simulink model "Md62StEnCtrl"  (R2018b)
settings: Solver=FixedStepDiscrete  StartTime=0.0  StopTime=10.0  RelTol=1e-3
undefined symbols (not defined in the file or in its folder): data, KeSMSuFirstRwStBackPosDelta_Val, KeSMSuThrdRwCushFoldPosDelta_Val, KeSMSwAcsMd30PassStFldUpwdDnwdPos1_Val, KeSMSwAcsMd30PassStFrwdBkwdPos1_Val, KeSMSwAcsMd31PassStBkReclnUpwdDnwdPos1_Val, KeSMSwSeatBkLimitPos_Val, KeSMSwSeatBkLimitPosDelt_Val, PassStBkReclnEn_Clear, PassStBkReclnEn_Set, PassStCshnFldEn_Clear, PassStCshnFldEn_Set, PassStFwdBkwdEn_Clear, PassStFwdBkwdEn_Set, SecRwLtStBkReclnEn_Clear, SecRwLtStBkReclnEn_Set, SecRwLtStFwdBkwdEn_Clear, SecRwLtStFwdBkwdEn_Set, SecRwLtStLgrstInwdOtwdEn_Clear, SecRwLtStLgrstInwdOtwdEn_Set, SecRwLtStLgrstUpwdDnwdEn_Clear, SecRwLtStLgrstUpwdDnwdEn_Set, SecRwRtStBkReclnEn_Clear, SecRwRtStBkReclnEn_Set, SecRwRtStFwdBkwdEn_Clear, SecRwRtStFwdBkwdEn_Set, SecRwRtStLgrstInwdOtwdEn_Clear, SecRwRtStLgrstInwdOtwdEn_Set, SecRwRtStLgrstUpwdDnwdEn_Clear, SecRwRtStLgrstUpwdDnwdEn_Set, ThdRwLtStBkReclnEn_Clear, ThdRwLtStBkReclnEn_Set, ThdRwLtStCshnFldEn_Clear, ThdRwLtStCshnFldEn_Set, ThdRwLtStFwdBkwdEn_Clear, ThdRwLtStFwdBkwdEn_Set, ThdRwRtStBkReclnEn_Clear, ThdRwRtStBkReclnEn_Set, ThdRwRtStCshnFldEn_Clear, ThdRwRtStCshnFldEn_Set, ThdRwRtStFwdBkwdEn_Clear, ThdRwRtStFwdBkwdEn_Set, ZeroLEn_Clear, ZeroLEn_Set, ZeroREn_Clear, ZeroREn_Set
libraries: simulink x1
(part 3 of 3)

== system Md62StEnCtrl/Md62StEnCtrl_Cal_sys/Subsystem/ThdRwRtStFwdBkwd_Clear ==
  note: Delete block
  MdBitNum : Inport
  Action Port : ActionPort  ActionType=else
  ThdRwRtStFwdBkwdEn_Clear : FunctionCaller  FunctionPrototype=ThdRwRtStFwdBkwdEn_Clear(data)  InputArgumentSpecifications=uint8(1)
  wires:
  MdBitNum/1 -> ThdRwRtStFwdBkwdEn_Clear/1

== system Md62StEnCtrl/Md62StEnCtrl_Cal_sys/Subsystem/ThdRwRtStFwdBkwd_Set ==
  note: Delete block
  MdBitNum : Inport
  Action Port : ActionPort  ActionType=then
  ThdRwRtStFwdBkwdEn_Set : FunctionCaller  FunctionPrototype=ThdRwRtStFwdBkwdEn_Set(data)  InputArgumentSpecifications=uint8(1)
  wires:
  MdBitNum/1 -> ThdRwRtStFwdBkwdEn_Set/1

== system Md62StEnCtrl/Md62StEnCtrl_Cal_sys/Subsystem/ZeroL_Clear ==
  note: Delete block
  MdBitNum : Inport
  Action Port : ActionPort  ActionType=else
  ZeroLEn_Clear : FunctionCaller  FunctionPrototype=ZeroLEn_Clear(data)  InputArgumentSpecifications=uint8(1)
  wires:
  MdBitNum/1 -> ZeroLEn_Clear/1

== system Md62StEnCtrl/Md62StEnCtrl_Cal_sys/Subsystem/ZeroL_Set ==
  note: Delete block
  MdBitNum : Inport
  Action Port : ActionPort  ActionType=then
  ZeroLEn_Set : FunctionCaller  FunctionPrototype=ZeroLEn_Set(data)  InputArgumentSpecifications=uint8(1)
  wires:
  MdBitNum/1 -> ZeroLEn_Set/1

== system Md62StEnCtrl/Md62StEnCtrl_Cal_sys/Subsystem/ZeroR_Clear ==
  note: Delete block
  MdBitNum : Inport
  Action Port : ActionPort  ActionType=else
  ZeroREn_Clear : FunctionCaller  FunctionPrototype=ZeroREn_Clear(data)  InputArgumentSpecifications=uint8(1)
  wires:
  MdBitNum/1 -> ZeroREn_Clear/1

== system Md62StEnCtrl/Md62StEnCtrl_Cal_sys/Subsystem/ZeroR_Set ==
  note: Delete block
  MdBitNum : Inport
  Action Port : ActionPort  ActionType=then
  ZeroREn_Set : FunctionCaller  FunctionPrototype=ZeroREn_Set(data)  InputArgumentSpecifications=uint8(1)
  wires:
  MdBitNum/1 -> ZeroREn_Set/1

== stateflow chart Md62StEnCtrl/Md62StEnCtrl_Cal_sys/Subsystem/Chart ==
  (default) -> (junction 20) : {
      | PassStBkReclnEn = 0;
      | PassStCshnFldEn = 0;
      | PassStFwdBkwdEn=0;
      | SecRwLtStBkReclnEn=0;
      | SecRwLtStFwdBkwdEn=0;
      | SecRwLtStLgrstInwdOtwdEn=0;
      | SecRwLtStLgrstUpwdDnwdEn=0;
      | SecRwRtStBkReclnEn=0;
      | SecRwRtStFwdBkwdEn=0;
      | SecRwRtStLgrstInwdOtwdEn=0;
      | SecRwRtStLgrstUpwdDnwdEn=0;
      | ThdRwLtStBkReclnEn=0;
      | ThdRwLtStCshnFldEn=0;
      | ThdRwLtStFwdBkwdEn=0;
      | ThdRwRtStBkReclnEn=0;
      | ThdRwRtStCshnFldEn=0;
      | ThdRwRtStFwdBkwdEn=0;
      | ZeroLEn=0;
      | ZeroREn=0;
      | PassStFwdBkwdFailflg = 0;
      | PassStCshnFldFailflg = 0;
      | }
  (junction 20) -> (junction 22) [order 1] : [!Stage1SecRwDone]
  (junction 22) -> (junction 26) [order 1] : [Md61ThdRwNotNeedFldOpn]
  (junction 20) -> (junction 44) [order 2]
  (junction 22) -> (junction 37) [order 2]
  (junction 26) -> (junction 28) : {
      | SecRwRtStLgrstInwdOtwdEn=1;
      | SecRwRtStLgrstUpwdDnwdEn=1;
      | }
  (junction 37) -> (junction 39) [order 1] : [Md61ThdRwLtStNotNeedFldOpn]
  (junction 39) -> (junction 499) [order 1] : [!SecRwRtStBkReclnStgDone ||...
      | !SecRwRtStLgrstOtwdInwdStgDone ||...
      | !SecRwRtStLgrstUpwdDnwdStgDone]
  (junction 44) -> (junction 46) [order 1] : [ThdRwLtNeedFld]
  (junction 46) -> (junction 52) [order 1] : [!ThdRwLtStBkReclnStgDone||!ThdRwLtStFwdBkwdStgDone]
  (junction 37) -> (junction 504) [order 2]
  (junction 39) -> (junction 41) [order 2] : {
      | SecRwRtStFwdBkwdEn=1;
      | }
  (junction 499) -> (junction 501) : {SecRwRtStLgrstInwdOtwdEn=1;
      | SecRwRtStLgrstUpwdDnwdEn=1;
      | SecRwRtStBkReclnEn=1;}
  (junction 44) -> (junction 71) [order 2]
  (junction 46) -> (junction 64) [order 2]
  (junction 52) -> (junction 56) : {
      | ThdRwLtStBkReclnEn = 1;
      | ThdRwLtStFwdBkwdEn=1;
      | }
  (junction 64) -> (junction 66) [order 1] : [!ThdRwLtStCshnFldStgDone]
  (junction 64) -> (junction 54) [order 2]
  (junction 66) -> (junction 68) : {
      | ThdRwLtStCshnFldEn=1;
      | }
  (junction 504) -> (junction 506) [order 1] : [!SecRwRtStBkReclnStgDone ||...
      | !SecRwRtStLgrstOtwdInwdStgDone ||...
      | !SecRwRtStLgrstUpwdDnwdStgDone]
  (junction 504) -> (junction 510) [order 2] : {SecRwRtStFwdBkwdEn=1;}
  (junction 506) -> (junction 508) : {SecRwRtStLgrstInwdOtwdEn=1;
      | SecRwRtStLgrstUpwdDnwdEn=1;
      | SecRwRtStBkReclnEn=1;}
  (junction 68) -> (junction 54)
  (junction 56) -> (junction 68)
  (junction 54) -> (junction 71)
  (junction 71) -> (junction 74)
  (junction 508) -> (junction 510)
  (junction 74) -> (junction 76) [order 1] : [ThdRwLtNeedOpn]
  (junction 76) -> (junction 78) [order 1] : [!ThdRwLtStCshnFldStgDone]
  (junction 510) -> (junction 513)
  (junction 74) -> (junction 92) [order 2]
  (junction 76) -> (junction 84) [order 2]
  (junction 78) -> (junction 80) : {
      | ThdRwLtStCshnFldEn=1;
      | }
  (junction 84) -> (junction 87) [order 1] : [!ThdRwLtStBkReclnStgDone||!ThdRwLtStFwdBkwdStgDone]
  (junction 84) -> (junction 82) [order 2]
  (junction 87) -> (junction 89) : {
      | ThdRwLtStBkReclnEn = 1;
      | ThdRwLtStFwdBkwdEn=1;
      | }
  (junction 513) -> (junction 515) [order 1] : [!SecRwLtStBkReclnStgDone ||...
      | !SecRwLtStLgrstOtwdInwdStgDone ||...
      | !SecRwLtStLgrstUpwdDnwdStgDone]
  (junction 513) -> (junction 30) [order 2] : {
      | SecRwLtStFwdBkwdEn=1;
      | }
  (junction 515) -> (junction 517) : {SecRwLtStBkReclnEn=1;
      | SecRwLtStLgrstInwdOtwdEn=1;
      | SecRwLtStLgrstUpwdDnwdEn=1;}
  (junction 82) -> (junction 92)
  (junction 89) -> (junction 82)
  (junction 80) -> (junction 89)
  (junction 92) -> (junction 95)
  (junction 95) -> (junction 121) [order 1] : [ThdRwRtNeedFld]
  (junction 121) -> (junction 124) [order 1] : [!ThdRwRtStBkReclnStgDone||!ThdRwRtStFwdBkwdStgDone]
  (junction 95) -> (junction 133) [order 2]
  (junction 121) -> (junction 119) [order 2]
  (junction 124) -> (junction 125) : {
      | ThdRwRtStBkReclnEn = 1;
      | ThdRwRtStFwdBkwdEn=1;
      | }
  (junction 119) -> (junction 128) [order 1] : [!ThdRwRtStCshnFldStgDone]
  (junction 119) -> (junction 130) [order 2]
  (junction 128) -> (junction 112) : {
      | ThdRwRtStCshnFldEn=1;
      | }
  (junction 130) -> (junction 133)
  (junction 112) -> (junction 130)
  (junction 125) -> (junction 112)
  (junction 133) -> (junction 135)
  (junction 135) -> (junction 109) [order 1] : [ThdRwRtNeedOpn]
  (junction 109) -> (junction 122) [order 1] : [!ThdRwRtStCshnFldStgDone]
  (junction 135) -> (junction 137) [order 2]
  (junction 109) -> (junction 114) [order 2]
  (junction 122) -> (junction 127) : {
      | ThdRwRtStCshnFldEn=1;
      | }
  (junction 114) -> (junction 104) [order 1] : [!ThdRwRtStBkReclnStgDone||!ThdRwRtStFwdBkwdStgDone]
  (junction 114) -> (junction 117) [order 2]
  (junction 104) -> (junction 106) : {
      | ThdRwRtStBkReclnEn = 1;
      | ThdRwRtStFwdBkwdEn=1;
      | }
  (junction 117) -> (junction 137)
  (junction 106) -> (junction 117)
  (junction 127) -> (junction 106)
  (junction 137) -> (junction 143)
  (junction 145) -> (junction 151) [order 1] : [PassStFwdBkwdStgDone ]
  (junction 143) -> (junction 145) [order 1] : [PassStNeedFld]
  (junction 151) -> (junction 152)
  (junction 143) -> (junction 33) [order 2]
  (junction 145) -> (junction 161) [order 2] : {PassStFwdBkwdEn = 1;}
  (junction 152) -> (junction 161)
  (junction 161) -> (junction 162)
  (junction 162) -> (junction 149) [order 1] : [ PassStBkReclnStgDone||(!PassStFwdBkwdStgDone&&PassStBkReclnUpwdDnwdPos<Md30PassStBkReclnTrgtPos1) ]
  (junction 162) -> (junction 163) [order 2] : {PassStBkReclnEn = 1;}
  (junction 149) -> (junction 150)
  (junction 150) -> (junction 163)
  (junction 163) -> (junction 167)
  (junction 167) -> (junction 168) [order 1] : [PassStFwdBkwdStgDone &&...
      | PassStFwdBkwdPos<(PassStFwdBkwdTrgtPos1-120)&&((PassStFldUpwdDnwdPos >PassStCshnFldTrgtPos1)||PassStBkReclnUpwdDnwdPos>120)]
  (junction 167) -> (junction 175) [order 2]
  (junction 168) -> (junction 173) : {PassStFwdBkwdFailflg =1;}
  (junction 173) -> (junction 175)
  (junction 175) -> (junction 184)
  (junction 184) -> (junction 187) [order 1] : [PassStFwdBkwdPos>=(PassStFwdBkwdTrgtPos1-120)]
  (junction 187) -> (junction 189) [order 1] : [PassStCshnFldStgDone ]
  (junction 189) -> (junction 172) [order 1] : [PassStFldUpwdDnwdPos >PassStCshnFldTrgtPos1]
  (junction 184) -> (junction 182) [order 2]
  (junction 187) -> (junction 174) [order 2] : {
      | PassStCshnFldEn = 1;
      | }
  (junction 189) -> (junction 176) [order 2]
  (junction 172) -> (junction 188) : {
      | PassStCshnFldFailflg = 1;
      | }
  (junction 182) -> (junction 33)
  (junction 174) -> (junction 182)
  (junction 176) -> (junction 174)
  (junction 188) -> (junction 176)
  (junction 33) -> (junction 204)
  (junction 204) -> (junction 206) [order 1] : [PassStNeedOpn]
  (junction 206) -> (junction 212) [order 1] : [PassStFwdBkwdStgDone ]
  (junction 212) -> (junction 213) [order 1] : [(PassStFwdBkwdPos<(PassStFwdBkwdTrgtPos1-120))&&...
      | (PassStBkReclnUpwdDnwdPos<Md61PassStBkReclnTrgtPos)]
  (junction 204) -> (junction 249) [order 2]
  (junction 206) -> (junction 243) [order 2] : {PassStFwdBkwdEn = 1;}
  (junction 212) -> (junction 208) [order 2]
  (junction 213) -> (junction 209) : {PassStFwdBkwdFailflg =1;}
  (junction 209) -> (junction 208)
  (junction 208) -> (junction 243)
  (junction 243) -> (junction 244)
  (junction 244) -> (junction 210) [order 1] : [PassStFwdBkwdStgDone &&...
      | (PassStFwdBkwdPos>=(PassStFwdBkwdTrgtPos1-120))]
  (junction 210) -> (junction 211) [order 1] : [PassStBkReclnStgDone ]
  (junction 211) -> (junction 214) [order 1] : [PassStBkReclnUpwdDnwdPos <Md31PassStBkReclnTrgtPos1]
  (junction 244) -> (junction 246) [order 2]
  (junction 210) -> (junction 220) [order 2] : {
      | PassStBkReclnEn = 1;
      | }
  (junction 211) -> (junction 219) [order 2]
  (junction 214) -> (junction 234) : {
      | PassStCshnFldFailflg = 1;
      | }
  (junction 219) -> (junction 220)
  (junction 220) -> (junction 217)
  (junction 217) -> (junction 215) [order 1] : [(PassStBkReclnUpwdDnwdPos >=Md31PassStBkReclnTrgtPos1)&&!PassStCshnFldStgDone]
  (junction 217) -> (junction 216) [order 2]
  (junction 215) -> (junction 218) : {PassStCshnFldEn = 1;}
  (junction 246) -> (junction 249)
  (junction 216) -> (junction 246)
  (junction 218) -> (junction 216)
  (junction 234) -> (junction 218)
  (junction 249) -> (junction 254)
  (junction 30) -> (junction 254)
  (junction 517) -> (junction 30)
  (junction 41) -> (junction 517)
  (junction 501) -> (junction 41)
  (junction 28) -> (junction 501)
  (junction 254) -> (junction 257)
  (junction 257) -> (junction 259) [order 1] : [Stage2Done]
  (junction 259) -> (junction 264) [order 1] : [Stage3ThdRwLtEn&&(!ThdRwLtStBkReclnStgDone||!ThdRwLtStFwdBkwdStgDone)]
  (junction 257) -> (junction 261) [order 2]
  (junction 259) -> (junction 282) [order 2]
  (junction 264) -> (junction 280) : {
      | ThdRwLtStBkReclnEn = 1;
      | ThdRwLtStFwdBkwdEn=1;
      | }
  (junction 280) -> (junction 282)
  (junction 282) -> (junction 272)
  (junction 272) -> (junction 274) [order 1] : [Stage3ThdRwRtEn&&(!ThdRwRtStBkReclnStgDone||!ThdRwRtStFwdBkwdStgDone)]
  (junction 272) -> (junction 287) [order 2]
  (junction 274) -> (junction 285) : {
      | ThdRwRtStBkReclnEn = 1;
      | ThdRwRtStFwdBkwdEn=1;
      | }
  (junction 285) -> (junction 287)
  (junction 287) -> (junction 276)
  (junction 276) -> (junction 278) [order 1] : [Stage3PassStFwdBkwdEn&&!PassStFwdBkwdStgDone]
  (junction 276) -> (junction 290) [order 2]
  (junction 278) -> (junction 292) : {PassStFwdBkwdEn = 1;}
  (junction 292) -> (junction 290)
  (junction 290) -> (junction 297)
  (junction 297) -> (junction 299) [order 1] : [Stage3PassStBkEn&&!PassStBkReclnStgDone]
  (junction 297) -> (junction 303) [order 2]
  (junction 299) -> (junction 301) : {PassStBkReclnEn = 1;}
  (junction 303) -> (junction 261)
  (junction 301) -> (junction 303)
  (junction 261) -> (junction 313)
  (junction 313) -> (junction 325) [order 1] : [Stage2Done&& Stage3Done]
  (junction 325) -> (junction 319) [order 1] : [IfVeSMSuSecRwLtStBkReclnUpwdDnwdPos>Ltbktrgt&&!SecRwLtStBkReclnStgDone]
  (junction 313) -> (junction 317) [order 2]
  (junction 325) -> (junction 332) [order 2]
  (junction 319) -> (junction 326) : {SecRwLtStBkReclnEn = 1;}
  (junction 326) -> (junction 332)
  (junction 332) -> (junction 322)
  (junction 322) -> (junction 321) [order 1] : [IfVeSMSuSecRwLtStLgrstOtwdInwdPos >Ltlgrstintrgt &&!SecRwLtStLgrstOtwdInwdStgDone]
  (junction 322) -> (junction 333) [order 2]
  (junction 321) -> (junction 320) : {SecRwLtStLgrstInwdOtwdEn = 1;}
  (junction 320) -> (junction 333)
  (junction 333) -> (junction 323)
  (junction 323) -> (junction 327) [order 1] : [IfVeSMSuSecRwLtStLgrstUpwdDnwdPos >Ltlgrstuptrgt && !SecRwLtStLgrstUpwdDnwdStgDone]
  (junction 323) -> (junction 328) [order 2]
  (junction 327) -> (junction 329) : {SecRwLtStLgrstUpwdDnwdEn = 1;}
  (junction 329) -> (junction 328)
  (junction 328) -> (junction 330)
  (junction 330) -> (junction 324) [order 1] : [IfVeSMSuSecRwLtStZeroPos >Ltzerotrgt && !ZeroLStgDone]
  (junction 330) -> (junction 331) [order 2]
  (junction 324) -> (junction 338) : {ZeroLEn = 1;}
  (junction 338) -> (junction 331)
  (junction 331) -> (junction 335)
  (junction 335) -> (junction 346) [order 1] : [(IfVeSMSuSecRwLtStBkReclnUpwdDnwdPos<=Ltbktrgt||SecRwLtStBkReclnStgDone)&&...
      | (IfVeSMSuSecRwLtStLgrstOtwdInwdPos <=Ltlgrstintrgt ||SecRwLtStLgrstOtwdInwdStgDone) &&...
      | (IfVeSMSuSecRwLtStLgrstUpwdDnwdPos <=Ltlgrstuptrgt ||SecRwLtStLgrstUpwdDnwdStgDone)&&...
      | (IfVeSMSuSecRwLtStZeroPos <= Ltzerotrgt || ZeroLStgDone)]
  (junction 346) -> (junction 340) [order 1] : [SecRwLtStFrwdBkwdStgDone]
  (junction 340) -> (junction 347) [order 1] : [SecRwLtStBkReclnStgDone]
  (junction 335) -> (junction 341) [order 2]
  (junction 346) -> (junction 343) [order 2] : {SecRwLtStFwdBkwdEn =1;}
  (junction 340) -> (junction 334) [order 2] : {SecRwLtStBkReclnEn = 1;}
  (junction 347) -> (junction 339)
  (junction 339) -> (junction 334)
  (junction 334) -> (junction 336)
  (junction 336) -> (junction 344) [order 1] : [ZeroLStgDone]
  (junction 336) -> (junction 342) [order 2] : {ZeroLEn = 1;}
  (junction 344) -> (junction 337)
  (junction 337) -> (junction 342)
  (junction 342) -> (junction 345) : {
      | SecRwLtStLgrstInwdOtwdEn=1;
      | SecRwLtStLgrstUpwdDnwdEn=1;
      | }
  (junction 343) -> (junction 341)
  (junction 345) -> (junction 343)
  (junction 341) -> (junction 404)
  (junction 404) -> (junction 410) [order 1] : [IfVeSMSuSecRwRtStBkReclnUpwdDnwdPos>Rtbktrgt&&!SecRwRtStBkReclnStgDone]
  (junction 404) -> (junction 406) [order 2]
  (junction 410) -> (junction 398) : {SecRwRtStBkReclnEn = 1;}
  (junction 398) -> (junction 406)
  (junction 406) -> (junction 400)
  (junction 400) -> (junction 388) [order 1] : [IfVeSMSuSecRwRtStLgrstOtwdInwdPos >Rtlgrstintrgt &&!SecRwRtStLgrstOtwdInwdStgDone]
  (junction 400) -> (junction 408) [order 2]
  (junction 388) -> (junction 390) : {SecRwRtStLgrstInwdOtwdEn = 1;}
  (junction 390) -> (junction 408)
  (junction 408) -> (junction 392)
  (junction 392) -> (junction 393) [order 1] : [IfVeSMSuSecRwRtStLgrstUpwdDnwdPos >Rtlgrstuptrgt && !SecRwRtStLgrstUpwdDnwdStgDone]
  (junction 392) -> (junction 413) [order 2]
  (junction 393) -> (junction 394) : {SecRwRtStLgrstUpwdDnwdEn = 1;}
  (junction 394) -> (junction 413)
  (junction 413) -> (junction 397)
  (junction 397) -> (junction 401) [order 1] : [IfVeSMSuSecRwRtStZeroPos >Rtzerotrgt && !ZeroRStgDone]
  (junction 397) -> (junction 411) [order 2]
  (junction 401) -> (junction 403) : {ZeroREn = 1; }
  (junction 403) -> (junction 411)
  (junction 411) -> (junction 402)
  (junction 402) -> (junction 389) [order 1] : [
      | (IfVeSMSuSecRwRtStBkReclnUpwdDnwdPos<=Rtbktrgt||SecRwRtStBkReclnStgDone)&&...
      | (IfVeSMSuSecRwRtStLgrstOtwdInwdPos <=Rtlgrstintrgt ||SecRwRtStLgrstOtwdInwdStgDone) &&...
      | (IfVeSMSuSecRwRtStLgrstUpwdDnwdPos <=Rtlgrstuptrgt ||SecRwRtStLgrstUpwdDnwdStgDone)&&...
      | (IfVeSMSuSecRwRtStZeroPos <=Rtzerotrgt || ZeroRStgDone)
      | ]
  (junction 389) -> (junction 391) [order 1] : [SecRwRtStFrwdBkwdStgDone]
  (junction 391) -> (junction 412) [order 1] : [SecRwRtStBkReclnStgDone]
  (junction 402) -> (junction 386) [order 2]
  (junction 389) -> (junction 399) [order 2] : {SecRwRtStFwdBkwdEn =1;}
  (junction 391) -> (junction 387) [order 2] : {SecRwRtStBkReclnEn = 1;}
  (junction 412) -> (junction 409)
  (junction 409) -> (junction 387)
  (junction 387) -> (junction 395)
  (junction 395) -> (junction 405) [order 1] : [ZeroRStgDone]
  (junction 395) -> (junction 407) [order 2] : {ZeroREn = 1; }
  (junction 405) -> (junction 385)
  (junction 385) -> (junction 407)
  (junction 407) -> (junction 396) : {
      | SecRwRtStLgrstInwdOtwdEn=1;
      | SecRwRtStLgrstUpwdDnwdEn=1;
      | }
  (junction 386) -> (junction 317)
  (junction 399) -> (junction 386)
  (junction 396) -> (junction 399)
  (junction 317) -> (junction 454)
  (junction 454) -> (junction 456) [order 1] : [Stage2Done&& Stage3Done&Stage4Done]
  (junction 454) -> (junction 462) [order 2]
  (junction 456) -> (junction 460) : {
      | ThdRwLtStBkReclnEn = 1;
      | ThdRwLtStFwdBkwdEn=1;
      | ThdRwRtStBkReclnEn = 1;
      | ThdRwRtStFwdBkwdEn=1;
      | PassStBkReclnEn = 1;
      | PassStFwdBkwdEn=1;
      | PassStCshnFldEn=1;
      | }
  (junction 460) -> (junction 462)
  data: PassStBkReclnEn output boolean; PassStCshnFldEn output boolean; PassStFwdBkwdEn output boolean; SecRwLtStBkReclnEn output boolean; SecRwLtStFwdBkwdEn output boolean; SecRwLtStLgrstInwdOtwdEn output boolean; SecRwLtStLgrstUpwdDnwdEn output boolean; SecRwRtStBkReclnEn output boolean; SecRwRtStFwdBkwdEn output boolean; SecRwRtStLgrstInwdOtwdEn output boolean; SecRwRtStLgrstUpwdDnwdEn output boolean; ThdRwLtStBkReclnEn output boolean; ThdRwLtStCshnFldEn output boolean; ThdRwLtStFwdBkwdEn output boolean; ThdRwRtStBkReclnEn output boolean; ThdRwRtStCshnFldEn output boolean; ThdRwRtStFwdBkwdEn output boolean; ZeroLEn output boolean; ZeroREn output boolean; Stage1SecRwDone input; Md61ThdRwNotNeedFldOpn input; Md61ThdRwLtStNotNeedFldOpn input; ThdRwLtNeedFld input; ThdRwRtNeedFld input; ThdRwLtNeedOpn input; ThdRwRtNeedOpn input; ThdRwLtStCshnFldStgDone input; ThdRwLtStBkReclnStgDone input; ThdRwRtStCshnFldStgDone input; ThdRwRtStBkReclnStgDone input; ThdRwLtStFwdBkwdStgDone input; ThdRwRtStFwdBkwdStgDone input; PassStNeedFld input; PassStNeedOpn input; PassStFwdBkwdStgDone input; PassStBkReclnStgDone input; PassStFwdBkwdFailflg output boolean; PassStBkReclnUpwdDnwdPos input; PassStCshnFldStgDone input; Md31PassStBkReclnTrgtPos1 input; PassStCshnFldTrgtPos1 input; PassStFwdBkwdTrgtPos1 input; PassStCshnFldFailflg output boolean; Stage2Done input; Stage3ThdRwLtEn input; Stage3ThdRwRtEn input; Stage3PassStFwdBkwdEn input; Stage3PassStBkEn input; Stage3Done input; Stage4Done input; IfVeSMSuSecRwLtStBkReclnUpwdDnwdPos input; IfVeSMSuSecRwLtStLgrstOtwdInwdPos input; IfVeSMSuSecRwLtStLgrstUpwdDnwdPos input; IfVeSMSuSecRwLtStZeroPos input; Ltbktrgt input; Ltlgrstintrgt input; Ltlgrstuptrgt input; Ltzerotrgt input; IfVeSMSuSecRwRtStBkReclnUpwdDnwdPos input; IfVeSMSuSecRwRtStLgrstOtwdInwdPos input; IfVeSMSuSecRwRtStLgrstUpwdDnwdPos input; IfVeSMSuSecRwRtStZeroPos input; Rtbktrgt input; Rtlgrstintrgt input; Rtlgrstuptrgt input; Rtzerotrgt input; SecRwLtStBkReclnStgDone input; ZeroLStgDone input; SecRwLtStFrwdBkwdStgDone input; SecRwLtStLgrstOtwdInwdStgDone input; SecRwLtStLgrstUpwdDnwdStgDone input; SecRwRtStBkReclnStgDone input; ZeroRStgDone input; SecRwRtStFrwdBkwdStgDone input; SecRwRtStLgrstOtwdInwdStgDone input; SecRwRtStLgrstUpwdDnwdStgDone input; Md30PassStBkReclnTrgtPos1 input; PassStFwdBkwdPos input; PassStFldUpwdDnwdPos input; Md61PassStBkReclnTrgtPos input
